simulink model "mut1_asof1945"  (R2015b)
settings: Solver=FixedStepDiscrete  StartTime=0.0  StopTime=200  FixedStep=1  RelTol=1e-3
undefined symbols (not defined in the file or in its folder): init
settings Model: Creator=swami  LastModifiedBy=shanku
settings DataIOCC: SaveFormat=Array
settings DebuggingCC: SolverPrmCheckMsg=warning
settings HardwareCC: ProdBitPerPointer=32  ProdLargestAtomicFloat=None  ProdIntDivRoundTo=Undefined  ProdEndianess=Unspecified  ProdWordSize=32  ProdHWDeviceType=32-bit Generic
settings GRTTargetCC: GeneratePreprocessorConditionals=Disable all
settings ConfigComp: CovModelRefEnable=Off  CovSFcnEnable=off

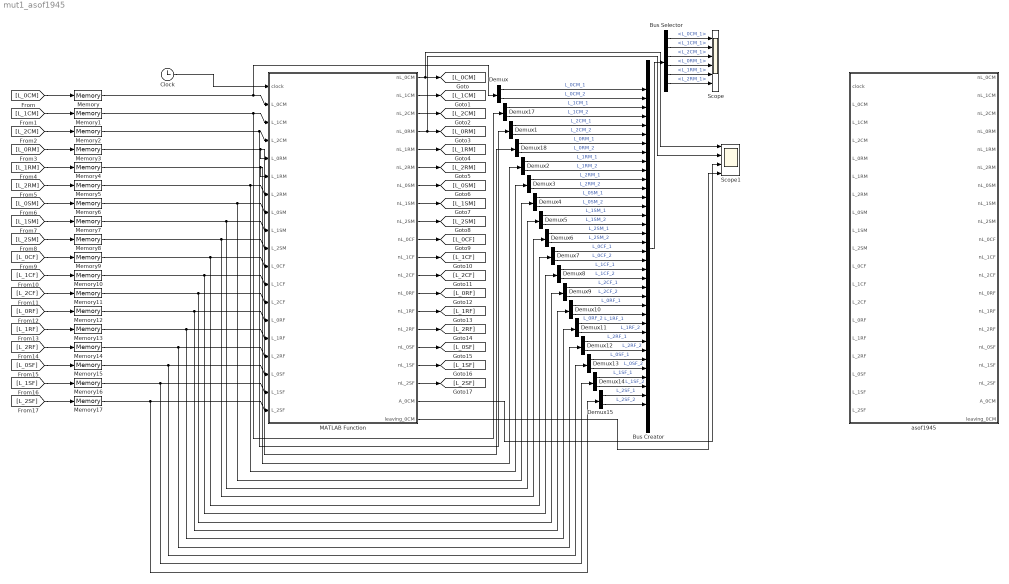
== system mut1_asof1945 ==
  Bus Creator : BusCreator  Inputs=36
  Bus Selector : BusSelector  OutputSignals=L_0CM_1,L_1CM_1,L_2CM_1,L_0RM_1,L_1RM_1,L_2RM_1
  Clock : Clock
  Demux{,1..15,17..18} (18 alike) : Demux  Outputs=2
  MATLAB Function : MATLAB Function  TreatAsAtomicUnit=on
  Memory : Memory  X0=init.L_0CM_0
  Memory1 : Memory  X0=init.L_1CM_0
  Memory10 : Memory  X0=init.L_1CF_0
  Memory11 : Memory  X0=init.L_2CF_0
  Memory12 : Memory  X0=init.L_0RF_0
  Memory13 : Memory  X0=init.L_1RF_0
  Memory14 : Memory  X0=init.L_2RF_0
  Memory15 : Memory  X0=init.L_0SF_0
  Memory16 : Memory  X0=init.L_1SF_0
  Memory17 : Memory  X0=init.L_2SF_0
  Memory2 : Memory  X0=init.L_2CM_0
  Memory3 : Memory  X0=init.L_0RM_0
  Memory4 : Memory  X0=init.L_1RM_0
  Memory5 : Memory  X0=init.L_2RM_0
  Memory6 : Memory  X0=init.L_0SM_0
  Memory7 : Memory  X0=init.L_1SM_0
  Memory8 : Memory  X0=init.L_2SM_0  LinearizeMemory=on
  Memory9 : Memory  X0=init.L_0CF_0
  Scope : Scope  NumInputPorts=6
  Scope1 : Scope  NumInputPorts=4
  asof1945 : MATLAB Function  TreatAsAtomicUnit=on
  wires:
  [L_1CM] -> Memory1/1
  [L_2CM] -> Memory2/1
  [L_0RM] -> Memory3/1
  [L_1RM] -> Memory4/1
  [L_2RM] -> Memory5/1
  [L_0SM] -> Memory6/1
  [L_1SM] -> Memory7/1
  [L_2SM] -> Memory8/1
  [L_0CF] -> Memory9/1
  [L_1CF] -> Memory10/1
  [L_2CF] -> Memory11/1
  [L_0RF] -> Memory12/1
  [L_1RF] -> Memory13/1
  [L_2RF] -> Memory14/1
  [L_0SF] -> Memory15/1
  [L_1SF] -> Memory16/1
  [L_2SF] -> Memory17/1
  MATLAB Function/12(nL_2CF) -> [L_2CF]
  MATLAB Function/13(nL_0RF) -> [L_0RF]
  MATLAB Function/14(nL_1RF) -> [L_1RF]
  MATLAB Function/15(nL_2RF) -> [L_2RF]
  MATLAB Function/1(nL_0CM) -> Scope1/1, [L_0CM]
  MATLAB Function/17(nL_1SF) -> [L_1SF]
  MATLAB Function/11(nL_1CF) -> [L_1CF]
  MATLAB Function/16(nL_0SF) -> [L_0SF]
  MATLAB Function/18(nL_2SF) -> [L_2SF]
  MATLAB Function/6(nL_2RM) -> [L_2RM]
  MATLAB Function/8(nL_1SM) -> [L_1SM]
  MATLAB Function/2(nL_1CM) -> [L_1CM]
  MATLAB Function/9(nL_2SM) -> [L_2SM]
  MATLAB Function/3(nL_2CM) -> [L_2CM]
  MATLAB Function/7(nL_0SM) -> [L_0SM]
  MATLAB Function/10(nL_0CF) -> [L_0CF]
  MATLAB Function/4(nL_0RM) -> Scope1/2, [L_0RM]
  MATLAB Function/5(nL_1RM) -> [L_1RM]
  Memory/1 -> Demux/1, MATLAB Function/2(L_0CM)
  Memory17/1 -> Demux15/1, MATLAB Function/19(L_2SF)
  Memory10/1 -> Demux8/1, MATLAB Function/12(L_1CF)
  Memory11/1 -> Demux9/1, MATLAB Function/13(L_2CF)
  Memory6/1 -> Demux4/1, MATLAB Function/8(L_0SM)
  Memory13/1 -> Demux11/1, MATLAB Function/15(L_1RF)
  Memory12/1 -> Demux10/1, MATLAB Function/14(L_0RF)
  Memory5/1 -> Demux3/1, MATLAB Function/7(L_2RM)
  Memory2/1 -> Demux1/1, MATLAB Function/4(L_2CM)
  Memory3/1 -> Demux18/1, MATLAB Function/5(L_0RM)
  Memory16/1 -> Demux14/1, MATLAB Function/18(L_1SF)
  Memory1/1 -> Demux17/1, MATLAB Function/3(L_1CM)
  Memory14/1 -> Demux12/1, MATLAB Function/16(L_2RF)
  Memory7/1 -> Demux5/1, MATLAB Function/9(L_1SM)
  Memory9/1 -> Demux7/1, MATLAB Function/11(L_0CF)
  Memory15/1 -> Demux13/1, MATLAB Function/17(L_0SF)
  Memory4/1 -> Demux2/1, MATLAB Function/6(L_1RM)
  [L_0CM] -> Memory/1
  Demux/1 -> Bus Creator/1  "L_0CM_1"
  Demux/2 -> Bus Creator/2  "L_0CM_2"
  Demux17/1 -> Bus Creator/3  "L_1CM_1"
  Demux17/2 -> Bus Creator/4  "L_1CM_2"
  Demux1/1 -> Bus Creator/5  "L_2CM_1"
  Demux1/2 -> Bus Creator/6  "L_2CM_2"
  Demux18/1 -> Bus Creator/7  "L_0RM_1"
  Demux18/2 -> Bus Creator/8  "L_0RM_2"
  Demux15/2 -> Bus Creator/36  "L_2SF_2"
  Demux15/1 -> Bus Creator/35  "L_2SF_1"
  Demux14/2 -> Bus Creator/34  "L_1SF_2"
  Demux14/1 -> Bus Creator/33  "L_1SF_1"
  Demux13/2 -> Bus Creator/32  "L_0SF_2"
  Demux13/1 -> Bus Creator/31  "L_0SF_1"
  Demux12/1 -> Bus Creator/29  "L_2RF_1"
  Demux12/2 -> Bus Creator/30  "L_2RF_2"
  Demux11/1 -> Bus Creator/27  "L_1RF_1"
  Demux11/2 -> Bus Creator/28  "L_1RF_2"
  Demux10/2 -> Bus Creator/26  "L_0RF_2"
  Demux10/1 -> Bus Creator/25  "L_0RF_1"
  Demux9/1 -> Bus Creator/23  "L_2CF_1"
  Demux9/2 -> Bus Creator/24  "L_2CF_2"
  Demux8/1 -> Bus Creator/21  "L_1CF_1"
  Demux8/2 -> Bus Creator/22  "L_1CF_2"
  Demux7/2 -> Bus Creator/20  "L_0CF_2"
  Demux7/1 -> Bus Creator/19  "L_0CF_1"
  Demux6/2 -> Bus Creator/18  "L_2SM_2"
  Demux6/1 -> Bus Creator/17  "L_2SM_1"
  Demux5/1 -> Bus Creator/15  "L_1SM_1"
  Demux5/2 -> Bus Creator/16  "L_1SM_2"
  Demux4/2 -> Bus Creator/14  "L_0SM_2"
  Demux4/1 -> Bus Creator/13  "L_0SM_1"
  Demux3/2 -> Bus Creator/12  "L_2RM_2"
  Demux3/1 -> Bus Creator/11  "L_2RM_1"
  Demux2/1 -> Bus Creator/9  "L_1RM_1"
  Demux2/2 -> Bus Creator/10  "L_1RM_2"
  Bus Creator/1 -> Bus Selector/1
  Bus Selector/1 -> Scope/1  "<L_0CM_1>"
  Bus Selector/2 -> Scope/2  "<L_1CM_1>"
  Bus Selector/3 -> Scope/3  "<L_2CM_1>"
  Bus Selector/4 -> Scope/4  "<L_0RM_1>"
  Bus Selector/5 -> Scope/5  "<L_1RM_1>"
  Bus Selector/6 -> Scope/6  "<L_2RM_1>"
  Memory8/1 -> Demux6/1, MATLAB Function/10(L_2SM)
  Clock/1 -> MATLAB Function/1(clock)
  MATLAB Function/19(A_0CM) -> Scope1/3
  MATLAB Function/20(leaving_0CM) -> Scope1/4

== matlab function mut1_asof1945/asof1945 ==
  data: clock input; L_0CM input; L_1CM input; L_2CM input; L_0RM input; L_1RM input; L_2RM input; L_0SM input; L_1SM input; L_2SM input; L_0CF input; L_1CF input; L_2CF input; L_0RF input; L_1RF input; L_2RF input; L_0SF input; L_1SF input; L_2SF input; nL_0CM output; nL_1CM output; nL_2CM output; nL_0RM output; nL_1RM output; nL_2RM output; nL_0SM output; nL_1SM output; nL_2SM output; nL_0CF output; nL_1CF output; nL_2CF output; nL_0RF output; nL_1RF output; nL_2RF output; nL_0SF output; nL_1SF output; nL_2SF output; mut parameter; A_0CM output; leaving_0CM output
function [nL_0CM, nL_1CM, nL_2CM, ...
          nL_0RM, nL_1RM, nL_2RM, ...
          nL_0SM, nL_1SM, nL_2SM, ...
          nL_0CF, nL_1CF, nL_2CF, ...
          nL_0RF, nL_1RF, nL_2RF, ...
          nL_0SF, nL_1SF, nL_2SF, ...
          A_0CM, leaving_0CM]   = fcn(...
          clock, L_0CM, L_1CM, L_2CM, ...
          L_0RM, L_1RM, L_2RM, ...
          L_0SM, L_1SM, L_2SM, ...
          L_0CF, L_1CF, L_2CF, ...
          L_0RF, L_1RF, L_2RF, ...
          L_0SF, L_1SF, L_2SF, ...
          mut)
if clock >= 35
    here=1;
end
% initialize sizes
nL_0CM = [0,0]; % first item is population size, second is cumulative age
nL_1CM = [0,0];
nL_2CM = [0,0];
nL_0CF = [0,0];
nL_1CF = [0,0];
nL_2CF = [0,0];
nL_0RM = [0,0];
nL_1RM = [0,0];
nL_2RM = [0,0];
nL_0RF = [0,0];
nL_1RF = [0,0];
nL_2RF = [0,0];
nL_0SM = [0,0];
nL_1SM = [0,0];
nL_2SM = [0,0];
nL_0SF = [0,0];
nL_1SF = [0,0];
nL_2SF = [0,0];
      
% calculate age by group
A_0CM = L_0CM(2) / L_0CM(1);
A_1CM = L_1CM(2) / L_1CM(1);
A_2CM = L_2CM(2) / L_2CM(1);
A_0CF = L_0CF(2) / L_0CF(1);
A_1CF = L_1CF(2) / L_1CF(1);
A_2CF = L_2CF(2) / L_2CF(1);
A_0RM = L_0RM(2) / L_0RM(1);
A_1RM = L_1RM(2) / L_1RM(1);
A_2RM = L_2RM(2) / L_2RM(1);
A_0RF = L_0RF(2) / L_0RF(1);
A_1RF = L_1RF(2) / L_1RF(1);
A_2RF = L_2RF(2) / L_2RF(1);
A_0SM = L_0SM(2) / L_0SM(1);
A_1SM = L_1SM(2) / L_1SM(1);
A_2SM = L_2SM(2) / L_2SM(1);
A_0SF = L_0SF(2) / L_0SF(1);
A_1SF = L_1SF(2) / L_1SF(1);
A_2SF = L_2SF(2) / L_2SF(1);

% calculate new children
[new_0CM, new_1CM, new_2CM, new_0CF, new_1CF, new_2CF] = ...
    getNewChildrenMutations( ...
          L_0RM, L_1RM, L_2RM, ...
          L_0RF, L_1RF, L_2RF, ...
          mut);


%calculate expiring population
expiring_0CM = 0;
expiring_1CM = 0;
expiring_2CM = 0;
expiring_0CF = 0;
expiring_1CF = 0;
expiring_2CF = 0;

expiring_0RM = 0;
expiring_1RM = 0;
expiring_2RM = 0;
expiring_0RF = 0;
expiring_1RF = 0;
expiring_2RF = 0;

expiring_0SM = 0.6 * L_0SM(1);
expiring_1SM = 0.6 * L_1SM(1);
expiring_2SM = 0.6 * L_2SM(1);
expiring_0SF = 0.4 * L_0SM(1);
expiring_1SF = 0.4 * L_1SM(1);
expiring_2SF = 0.4 * L_2SM(1);

% calculate movement between groups

leaving_0CM = min(max(L_0CM(2) - (L_0CM(1)-expiring_0CM) * mut.Y_C,0), ...
    (L_0CM(1)-expiring_0CM));
incoming_0RM = leaving_0CM;
leaving_1CM = min(max(L_1CM(2) - (L_1CM(1)-expiring_1CM) * mut.Y_C,0), ...
    L_1CM(1)-expiring_1CM);
incoming_1RM = leaving_1CM;
leaving_2CM = min(max(L_2CM(2) - (L_2CM(1)-expiring_2CM) * mut.Y_C,0), ...
    L_2CM(1)-expiring_2CM);
incoming_2RM = leaving_2CM;
leaving_0CF = min(max(L_0CF(2) - (L_0CF(1)-expiring_0CF) * mut.Y_C,0), ...
    L_0CF(1)-expiring_0CF);
incoming_0RF = leaving_0CF;
leaving_1CF = min(max(L_1CF(2) - (L_1CF(1)-expiring_1CF) * mut.Y_C,0), ...
    L_1CF(1)-expiring_1CF);
incoming_1RF = leaving_1CF;
leaving_2CF = min(max(L_2CF(2) - (L_2CF(1)-expiring_2CF) * mut.Y_C,0), ...
    L_2CF(1)-expiring_2CF);
incoming_2RF = leaving_2CF;

leaving_0RM = min(max(L_0RM(2) - (L_0RM(1)-expiring_0RM) * mut.Y_R,0), ...
    L_0RM(1)-expiring_0RM);
incoming_0SM = leaving_0RM;
leaving_1RM = min(max(L_1RM(2) - (L_1RM(1)-expiring_1RM) * mut.Y_R,0), ...
    L_1RM(1)-expiring_1RM);
incoming_1SM = leaving_1RM;
leaving_2RM = min(max(L_2RM(2) - (L_2RM(1)-expiring_2RM) * mut.Y_R,0), ...
    L_2RM(1)-expiring_2RM);
incoming_2SM = leaving_2RM;
leaving_0RF = min(max(L_0RF(2) - (L_0RF(1)-expiring_0RF) * mut.Y_R,0), ...
    L_0RF(1)-expiring_0RF);
incoming_0SF = leaving_0RF;
leaving_1RF = min(max(L_1RF(2) - (L_1RF(1)-expiring_1RF) * mut.Y_R,0), ...
    L_1RF(1)-expiring_1RF);
incoming_1SF = leaving_1RF;
leaving_2RF = min(max(L_2RF(2) - (L_2RF(1)-expiring_2RF) * mut.Y_R,0), ...
    L_2RF(1)-expiring_2RF);
incoming_2SF = leaving_2RF;

%POPULATION
% update population size for children
nL_0CM(1) = L_0CM(1) + new_0CM - leaving_0CM - expiring_0CM;
nL_1CM(1) = L_1CM(1) + new_1CM - leaving_1CM - expiring_1CM;
nL_2CM(1) = L_2CM(1) + new_2CM - leaving_2CM - expiring_2CM;
nL_0CF(1) = L_0CF(1) + new_0CF - leaving_0CF - expiring_0CF;
nL_1CF(1) = L_1CF(1) + new_1CF - leaving_1CF - expiring_1CF;
nL_2CF(1) = L_2CF(1) + new_2CF - leaving_2CF - expiring_2CF;

% update population size for reproducing adults
nL_0RM(1) = L_0RM(1) + incoming_0RM - leaving_0RM - expiring_0RM;
nL_1RM(1) = L_1RM(1) + incoming_1RM - leaving_1RM - expiring_1RM;
nL_2RM(1) = L_2RM(1) + incoming_2RM - leaving_2RM - expiring_2RM;
nL_0RF(1) = L_0RF(1) + incoming_0RF - leaving_0RF - expiring_0RF;
nL_1RF(1) = L_1RF(1) + incoming_1RF - leaving_1RF - expiring_1RF;
nL_2RF(1) = L_2RF(1) + incoming_2RF - leaving_2RF - expiring_2RF;

% update population size for senior adults
nL_0SM(1) = L_0SM(1) + incoming_0SM - expiring_0SM;
nL_1SM(1) = L_1SM(1) + incoming_1SM - expiring_1SM;
nL_2SM(1) = L_2SM(1) + incoming_2SM - expiring_2SM;
nL_0SF(1) = L_0SF(1) + incoming_0SF - expiring_0SF;
nL_1SF(1) = L_1SF(1) + incoming_1SF - expiring_1SF;
nL_2SF(1) = L_2SF(1) + incoming_2SF - expiring_2SF;

% update cumulative age of children
nL_0CM(2) = L_0CM(2) + L_0CM(1) - leaving_0CM * (mut.Y_C-1) - expiring_0CM * A_0CM;
nL_1CM(2) = L_1CM(2) + L_1CM(1) - leaving_1CM * (mut.Y_C-1) - expiring_1CM * A_1CM;
nL_2CM(2) = L_2CM(2) + L_2CM(1) - leaving_2CM * (mut.Y_C-1) - expiring_2CM * A_2CM;
nL_0CF(2) = L_0CF(2) + L_0CF(1) - leaving_0CF * (mut.Y_C-1) - expiring_0CF * A_0CF;
nL_1CF(2) = L_1CF(2) + L_1CF(1) - leaving_1CF * (mut.Y_C-1) - expiring_1CF * A_1CF;
nL_2CF(2) = L_2CF(2) + L_2CF(1) - leaving_2CF * (mut.Y_C-1) - expiring_2CF * A_2CF;


% update cumulative age of reproducing adults
nL_0RM(2) = L_0RM(2) + L_0RM(1) + incoming_0RM * (mut.Y_C+1) - leaving_0RM * (mut.Y_R-1) - expiring_0RM * A_0RM;
nL_1RM(2) = L_1RM(2) + L_1RM(1) + incoming_1RM * (mut.Y_C+1) - leaving_1RM * (mut.Y_R-1) - expiring_1RM * A_1RM;
nL_2RM(2) = L_2RM(2) + L_2RM(1) + incoming_2RM * (mut.Y_C+1) - leaving_2RM * (mut.Y_R-1) - expiring_2RM * A_2RM;
nL_0RF(2) = L_0RF(2) + L_0RF(1) + incoming_0RF * (mut.Y_C+1) - leaving_0RF * (mut.Y_R-1) - expiring_0RF * A_0RF;
nL_1RF(2) = L_1RF(2) + L_1RF(1) + incoming_1RF * (mut.Y_C+1) - leaving_1RF * (mut.Y_R-1) - expiring_1RF * A_1RF;
nL_2RF(2) = L_2RF(2) + L_2RF(1) + incoming_2RF * (mut.Y_C+1) - leaving_2RF * (mut.Y_R-1) - expiring_2RF * A_2RF;

% update cumulative age of senior adults
nL_0SM(2) = L_0SM(2) + L_0SM(1) + incoming_0SM * (mut.Y_R+1) - expiring_0SM * A_0SM;
nL_1SM(2) = L_1SM(2) + L_1SM(1) + incoming_1SM * (mut.Y_R+1) - expiring_1SM * A_1SM;
nL_2SM(2) = L_2SM(2) + L_2SM(1) + incoming_2SM * (mut.Y_R+1) - expiring_2SM * A_2SM;
nL_0SF(2) = L_0SF(2) + L_0SF(1) + incoming_0SF * (mut.Y_R+1) - expiring_0SF * A_0SF;
nL_1SF(2) = L_1SF(2) + L_1SF(1) + incoming_1SF * (mut.Y_R+1) - expiring_1SF * A_1SF;
nL_2SF(2) = L_2SF(2) + L_2SF(1) + incoming_2SF * (mut.Y_R+1) - expiring_2SF * A_2SF;


return

function [new_0CM, new_1CM, new_2CM, new_0CF, new_1CF, new_2CF] = ...
    getNewChildrenMutations( ...
          L_0RM, L_1RM, L_2RM, ...
          L_0RF, L_1RF, L_2RF, ...
          mut)

% calculte total populations
L_TRM = L_0RM(1) + L_1RM(1) + L_2RM(1);
L_TRF = L_0RF(1) + L_1RF(1) + L_2RF(1);


new_TC = mut.fertility * L_TRM * mut.fertility * L_TRF;
% NOTE: should I consider other models for the above?
new_TCM = new_TC * mut.M2Fprobability;
new_TCF = new_TC * (1 - mut.M2Fprobability);
      
% calculate probability of parents being of certain mutation type
probParents = eye(3);
probParents(1,1) = (L_0RM(1) / L_TRM) * (L_0RF(1) / L_TRF);
probParents(1,2) = (L_0RM(1) / L_TRM) * (L_1RF(1) / L_TRF);
probParents(1,3) = (L_0RM(1) / L_TRM) * (L_2RF(1) / L_TRF);

probParents(2,1) = (L_1RM(1) / L_TRM) * (L_0RF(1) / L_TRF);
probParents(2,2) = (L_1RM(1) / L_TRM) * (L_1RF(1) / L_TRF);
probParents(2,3) = (L_1RM(1) / L_TRM) * (L_2RF(1) / L_TRF);

probParents(3,1) = (L_2RM(1) / L_TRM) * (L_0RF(1) / L_TRF);
probParents(3,2) = (L_2RM(1) / L_TRM) * (L_1RF(1) / L_TRF);
probParents(3,3)= (L_2RM(1) / L_TRM) * (L_2RF(1) / L_TRF);

[p0, p1, p2] = probMutationInheritance;

new_0CM = sum(sum(probParents .* p0)) * new_TCM;
new_1CM = sum(sum(probParents .* p1)) * new_TCM;
new_2CM = sum(sum(probParents .* p2)) * new_TCM;
new_0CF = sum(sum(probParents .* p0)) * new_TCF;
new_1CF = sum(sum(probParents .* p1)) * new_TCF;
new_2CF = sum(sum(probParents .* p2)) * new_TCF;



return

function [p0, p1, p2] = probMutationInheritance

p0 = eye(3)*0;
p1 = eye(3)*0;
p2 = eye(3)*0;

p0(1,1) = 1.0;
p0(1,2) = 0.5;
p0(1,3) = 0.0;
p0(2,1) = 0.5;
p0(2,2) = 0.25;
p0(2,3) = 0.0;
p0(3,1) = 0.0;
p0(3,2) = 0.0;
p0(3,3) = 0.0;

p1(1,1) = 0.0;
p1(1,2) = 0.5;
p1(1,3) = 1.0;
p1(2,1) = 0.5;
p1(2,2) = 0.5;
p1(2,3) = 0.5;
p1(3,1) = 1.0;
p1(3,2) = 0.5;
p1(3,3) = 0.0;

p2(1,1) = 0.0;
p2(1,2) = 0.0;
p2(1,3) = 0.0;
p2(2,1) = 0.0;
p2(2,2) = 0.25;
p2(2,3) = 0.5;
p2(3,1) = 0.0;
p2(3,2) = 0.5;
p2(3,3) = 1.0;

return

== matlab function mut1_asof1945/MATLAB Function ==
  data: clock input; L_0CM input; L_1CM input; L_2CM input; L_0RM input; L_1RM input; L_2RM input; L_0SM input; L_1SM input; L_2SM input; L_0CF input; L_1CF input; L_2CF input; L_0RF input; L_1RF input; L_2RF input; L_0SF input; L_1SF input; L_2SF input; nL_0CM output; nL_1CM output; nL_2CM output; nL_0RM output; nL_1RM output; nL_2RM output; nL_0SM output; nL_1SM output; nL_2SM output; nL_0CF output; nL_1CF output; nL_2CF output; nL_0RF output; nL_1RF output; nL_2RF output; nL_0SF output; nL_1SF output; nL_2SF output; mut parameter; A_0CM output; leaving_0CM output
function [nL_0CM, nL_1CM, nL_2CM, ...
          nL_0RM, nL_1RM, nL_2RM, ...
          nL_0SM, nL_1SM, nL_2SM, ...
          nL_0CF, nL_1CF, nL_2CF, ...
          nL_0RF, nL_1RF, nL_2RF, ...
          nL_0SF, nL_1SF, nL_2SF, ...
          A_0CM, leaving_0CM]   = MutationModel(...
          clock, L_0CM, L_1CM, L_2CM, ...
          L_0RM, L_1RM, L_2RM, ...
          L_0SM, L_1SM, L_2SM, ...
          L_0CF, L_1CF, L_2CF, ...
          L_0RF, L_1RF, L_2RF, ...
          L_0SF, L_1SF, L_2SF, ...
          mut)
if clock >= 35
    here=1;
end
% initialize sizes
nL_0CM = [0,0]; % first item is population size, second is cumulative age
nL_1CM = [0,0];
nL_2CM = [0,0];
nL_0CF = [0,0];
nL_1CF = [0,0];
nL_2CF = [0,0];
nL_0RM = [0,0];
nL_1RM = [0,0];
nL_2RM = [0,0];
nL_0RF = [0,0];
nL_1RF = [0,0];
nL_2RF = [0,0];
nL_0SM = [0,0];
nL_1SM = [0,0];
nL_2SM = [0,0];
nL_0SF = [0,0];
nL_1SF = [0,0];
nL_2SF = [0,0];
      
% calculate age by group
A_0CM = L_0CM(2) / L_0CM(1);
A_1CM = L_1CM(2) / L_1CM(1);
A_2CM = L_2CM(2) / L_2CM(1);
A_0CF = L_0CF(2) / L_0CF(1);
A_1CF = L_1CF(2) / L_1CF(1);
A_2CF = L_2CF(2) / L_2CF(1);
A_0RM = L_0RM(2) / L_0RM(1);
A_1RM = L_1RM(2) / L_1RM(1);
A_2RM = L_2RM(2) / L_2RM(1);
A_0RF = L_0RF(2) / L_0RF(1);
A_1RF = L_1RF(2) / L_1RF(1);
A_2RF = L_2RF(2) / L_2RF(1);
A_0SM = L_0SM(2) / L_0SM(1);
A_1SM = L_1SM(2) / L_1SM(1);
A_2SM = L_2SM(2) / L_2SM(1);
A_0SF = L_0SF(2) / L_0SF(1);
A_1SF = L_1SF(2) / L_1SF(1);
A_2SF = L_2SF(2) / L_2SF(1);

% calculate new children
[new_0CM, new_1CM, new_2CM, new_0CF, new_1CF, new_2CF] = ...
    getNewChildrenMutations( ...
          L_0RM, L_1RM, L_2RM, ...
          L_0RF, L_1RF, L_2RF, ...
          mut);


%calculate expiring population
expiring_0CM = 0;
expiring_1CM = 0;
expiring_2CM = 0;
expiring_0CF = 0;
expiring_1CF = 0;
expiring_2CF = 0;

expiring_0RM = 0;
expiring_1RM = 0;
expiring_2RM = 0;
expiring_0RF = 0;
expiring_1RF = 0;
expiring_2RF = 0;

expiring_0SM = 0.6 * L_0SM(1);
expiring_1SM = 0.6 * L_1SM(1);
expiring_2SM = 0.6 * L_2SM(1);
expiring_0SF = 0.4 * L_0SM(1);
expiring_1SF = 0.4 * L_1SM(1);
expiring_2SF = 0.4 * L_2SM(1);

% calculate movement between groups

leaving_0CM = min(max(L_0CM(2) - (L_0CM(1)-expiring_0CM) * mut.Y_C,0), ...
    (L_0CM(1)-expiring_0CM));
incoming_0RM = leaving_0CM;
leaving_1CM = min(max(L_1CM(2) - (L_1CM(1)-expiring_1CM) * mut.Y_C,0), ...
    L_1CM(1)-expiring_1CM);
incoming_1RM = leaving_1CM;
leaving_2CM = min(max(L_2CM(2) - (L_2CM(1)-expiring_2CM) * mut.Y_C,0), ...
    L_2CM(1)-expiring_2CM);
incoming_2RM = leaving_2CM;
leaving_0CF = min(max(L_0CF(2) - (L_0CF(1)-expiring_0CF) * mut.Y_C,0), ...
    L_0CF(1)-expiring_0CF);
incoming_0RF = leaving_0CF;
leaving_1CF = min(max(L_1CF(2) - (L_1CF(1)-expiring_1CF) * mut.Y_C,0), ...
    L_1CF(1)-expiring_1CF);
incoming_1RF = leaving_1CF;
leaving_2CF = min(max(L_2CF(2) - (L_2CF(1)-expiring_2CF) * mut.Y_C,0), ...
    L_2CF(1)-expiring_2CF);
incoming_2RF = leaving_2CF;

leaving_0RM = min(max(L_0RM(2) - (L_0RM(1)-expiring_0RM) * mut.Y_R,0), ...
    L_0RM(1)-expiring_0RM);
incoming_0SM = leaving_0RM;
leaving_1RM = min(max(L_1RM(2) - (L_1RM(1)-expiring_1RM) * mut.Y_R,0), ...
    L_1RM(1)-expiring_1RM);
incoming_1SM = leaving_1RM;
leaving_2RM = min(max(L_2RM(2) - (L_2RM(1)-expiring_2RM) * mut.Y_R,0), ...
    L_2RM(1)-expiring_2RM);
incoming_2SM = leaving_2RM;
leaving_0RF = min(max(L_0RF(2) - (L_0RF(1)-expiring_0RF) * mut.Y_R,0), ...
    L_0RF(1)-expiring_0RF);
incoming_0SF = leaving_0RF;
leaving_1RF = min(max(L_1RF(2) - (L_1RF(1)-expiring_1RF) * mut.Y_R,0), ...
    L_1RF(1)-expiring_1RF);
incoming_1SF = leaving_1RF;
leaving_2RF = min(max(L_2RF(2) - (L_2RF(1)-expiring_2RF) * mut.Y_R,0), ...
    L_2RF(1)-expiring_2RF);
incoming_2SF = leaving_2RF;

%POPULATION
% update population size for children
nL_0CM(1) = L_0CM(1) + new_0CM - leaving_0CM - expiring_0CM;
nL_1CM(1) = L_1CM(1) + new_1CM - leaving_1CM - expiring_1CM;
nL_2CM(1) = L_2CM(1) + new_2CM - leaving_2CM - expiring_2CM;
nL_0CF(1) = L_0CF(1) + new_0CF - leaving_0CF - expiring_0CF;
nL_1CF(1) = L_1CF(1) + new_1CF - leaving_1CF - expiring_1CF;
nL_2CF(1) = L_2CF(1) + new_2CF - leaving_2CF - expiring_2CF;

% update population size for reproducing adults
nL_0RM(1) = L_0RM(1) + incoming_0RM - leaving_0RM - expiring_0RM;
nL_1RM(1) = L_1RM(1) + incoming_1RM - leaving_1RM - expiring_1RM;
nL_2RM(1) = L_2RM(1) + incoming_2RM - leaving_2RM - expiring_2RM;
nL_0RF(1) = L_0RF(1) + incoming_0RF - leaving_0RF - expiring_0RF;
nL_1RF(1) = L_1RF(1) + incoming_1RF - leaving_1RF - expiring_1RF;
nL_2RF(1) = L_2RF(1) + incoming_2RF - leaving_2RF - expiring_2RF;

% update population size for senior adults
nL_0SM(1) = L_0SM(1) + incoming_0SM - expiring_0SM;
nL_1SM(1) = L_1SM(1) + incoming_1SM - expiring_1SM;
nL_2SM(1) = L_2SM(1) + incoming_2SM - expiring_2SM;
nL_0SF(1) = L_0SF(1) + incoming_0SF - expiring_0SF;
nL_1SF(1) = L_1SF(1) + incoming_1SF - expiring_1SF;
nL_2SF(1) = L_2SF(1) + incoming_2SF - expiring_2SF;

% update cumulative age of children
nL_0CM(2) = L_0CM(2) + L_0CM(1) - leaving_0CM * (mut.Y_C+1) - expiring_0CM * A_0CM;
nL_1CM(2) = L_1CM(2) + L_1CM(1) - leaving_1CM * (mut.Y_C+1) - expiring_1CM * A_1CM;
nL_2CM(2) = L_2CM(2) + L_2CM(1) - leaving_2CM * (mut.Y_C+1) - expiring_2CM * A_2CM;
nL_0CF(2) = L_0CF(2) + L_0CF(1) - leaving_0CF * (mut.Y_C+1) - expiring_0CF * A_0CF;
nL_1CF(2) = L_1CF(2) + L_1CF(1) - leaving_1CF * (mut.Y_C+1) - expiring_1CF * A_1CF;
nL_2CF(2) = L_2CF(2) + L_2CF(1) - leaving_2CF * (mut.Y_C+1) - expiring_2CF * A_2CF;


% update cumulative age of reproducing adults
nL_0RM(2) = L_0RM(2) + L_0RM(1) + incoming_0RM * (mut.Y_C-1) - leaving_0RM * (mut.Y_R+1) - expiring_0RM * A_0RM;
nL_1RM(2) = L_1RM(2) + L_1RM(1) + incoming_1RM * (mut.Y_C-1) - leaving_1RM * (mut.Y_R+1) - expiring_1RM * A_1RM;
nL_2RM(2) = L_2RM(2) + L_2RM(1) + incoming_2RM * (mut.Y_C-1) - leaving_2RM * (mut.Y_R+1) - expiring_2RM * A_2RM;
nL_0RF(2) = L_0RF(2) + L_0RF(1) + incoming_0RF * (mut.Y_C-1) - leaving_0RF * (mut.Y_R+1) - expiring_0RF * A_0RF;
nL_1RF(2) = L_1RF(2) + L_1RF(1) + incoming_1RF * (mut.Y_C-1) - leaving_1RF * (mut.Y_R+1) - expiring_1RF * A_1RF;
nL_2RF(2) = L_2RF(2) + L_2RF(1) + incoming_2RF * (mut.Y_C-1) - leaving_2RF * (mut.Y_R+1) - expiring_2RF * A_2RF;

% update cumulative age of senior adults
nL_0SM(2) = L_0SM(2) + L_0SM(1) + incoming_0SM * (mut.Y_R-1) - expiring_0SM * A_0SM;
nL_1SM(2) = L_1SM(2) + L_1SM(1) + incoming_1SM * (mut.Y_R-1) - expiring_1SM * A_1SM;
nL_2SM(2) = L_2SM(2) + L_2SM(1) + incoming_2SM * (mut.Y_R-1) - expiring_2SM * A_2SM;
nL_0SF(2) = L_0SF(2) + L_0SF(1) + incoming_0SF * (mut.Y_R-1) - expiring_0SF * A_0SF;
nL_1SF(2) = L_1SF(2) + L_1SF(1) + incoming_1SF * (mut.Y_R-1) - expiring_1SF * A_1SF;
nL_2SF(2) = L_2SF(2) + L_2SF(1) + incoming_2SF * (mut.Y_R-1) - expiring_2SF * A_2SF;


return

function [new_0CM, new_1CM, new_2CM, new_0CF, new_1CF, new_2CF] = ...
    getNewChildrenMutations( ...
          L_0RM, L_1RM, L_2RM, ...
          L_0RF, L_1RF, L_2RF, ...
          mut)

% calculte total populations
L_TRM = L_0RM(1) + L_1RM(1) + L_2RM(1);
L_TRF = L_0RF(1) + L_1RF(1) + L_2RF(1);


new_TC = mut.fertility * L_TRM * mut.fertility * L_TRF;
% NOTE: should I consider other models for the above?
new_TCM = new_TC * mut.M2Fprobability;
new_TCF = new_TC * (1 - mut.M2Fprobability);
      
% calculate probability of parents being of certain mutation type
probParents = eye(3);
probParents(1,1) = (L_0RM(1) / L_TRM) * (L_0RF(1) / L_TRF);
probParents(1,2) = (L_0RM(1) / L_TRM) * (L_1RF(1) / L_TRF);
probParents(1,3) = (L_0RM(1) / L_TRM) * (L_2RF(1) / L_TRF);

probParents(2,1) = (L_1RM(1) / L_TRM) * (L_0RF(1) / L_TRF);
probParents(2,2) = (L_1RM(1) / L_TRM) * (L_1RF(1) / L_TRF);
probParents(2,3) = (L_1RM(1) / L_TRM) * (L_2RF(1) / L_TRF);

probParents(3,1) = (L_2RM(1) / L_TRM) * (L_0RF(1) / L_TRF);
probParents(3,2) = (L_2RM(1) / L_TRM) * (L_1RF(1) / L_TRF);
probParents(3,3)= (L_2RM(1) / L_TRM) * (L_2RF(1) / L_TRF);

[p0, p1, p2] = probMutationInheritance;

new_0CM = sum(sum(probParents .* p0)) * new_TCM;
new_1CM = sum(sum(probParents .* p1)) * new_TCM;
new_2CM = sum(sum(probParents .* p2)) * new_TCM;
new_0CF = sum(sum(probParents .* p0)) * new_TCF;
new_1CF = sum(sum(probParents .* p1)) * new_TCF;
new_2CF = sum(sum(probParents .* p2)) * new_TCF;



return

function [p0, p1, p2] = probMutationInheritance

p0 = eye(3)*0;
p1 = eye(3)*0;
p2 = eye(3)*0;

p0(1,1) = 1.0;
p0(1,2) = 0.5;
p0(1,3) = 0.0;
p0(2,1) = 0.5;
p0(2,2) = 0.25;
p0(2,3) = 0.0;
p0(3,1) = 0.0;
p0(3,2) = 0.0;
p0(3,3) = 0.0;

p1(1,1) = 0.0;
p1(1,2) = 0.5;
p1(1,3) = 1.0;
p1(2,1) = 0.5;
p1(2,2) = 0.5;
p1(2,3) = 0.5;
p1(3,1) = 1.0;
p1(3,2) = 0.5;
p1(3,3) = 0.0;

p2(1,1) = 0.0;
p2(1,2) = 0.0;
p2(1,3) = 0.0;
p2(2,1) = 0.0;
p2(2,2) = 0.25;
p2(2,3) = 0.5;
p2(3,1) = 0.0;
p2(3,2) = 0.5;
p2(3,3) = 1.0;

return
